simulink model "Non Augmented plant Nor Reference Non-constrained Input"  (R2013a)
settings: Solver=ode45  StartTime=0.0  StopTime=10.0  RelTol=1e-3
settings Model: Creator=G.force  LastModifiedBy=G.force

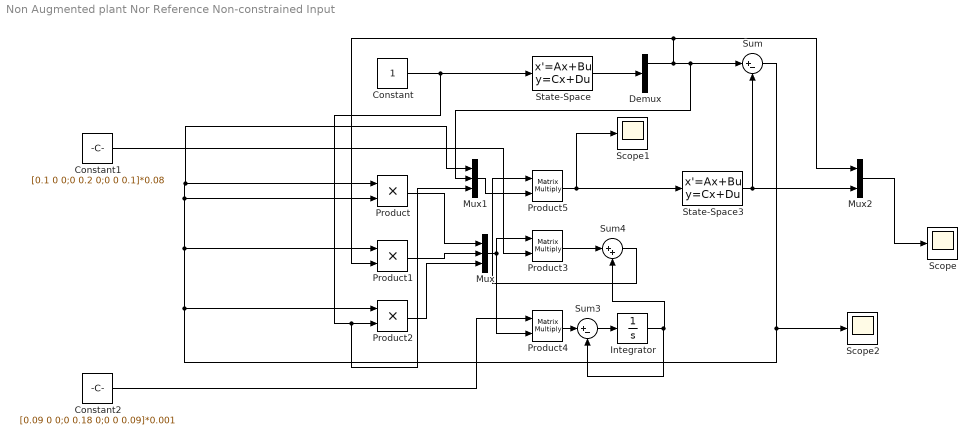
== system Non Augmented plant Nor Reference Non-constrained Input ==
  Constant : Constant
  Constant1 : Constant  Value=[0.1 0 0;0 0.2 0;0 0 0.1]*0.08
  Constant2 : Constant  Value=[0.09 0 0;0 0.18 0;0 0 0.09]*0.001
  Demux : Demux  Outputs=2
  Integrator : Integrator  InitialCondition=[0.01 0.0208 1e-6]
  Mux : Mux  Inputs=3
  Mux1 : Mux  Inputs=3
  Mux2 : Mux  Inputs=2
  Product : Product
  Product1 : Product
  Product2 : Product
  Product3 : Product  Multiplication=Matrix(*)
  Product4 : Product  Multiplication=Matrix(*)
  Product5 : Product  Multiplication=Matrix(*)
  Scope : Scope
      settings: ShowLegends=on  TimeRange=4  YMin=-40  YMax=45  SaveName=sd  MaxDataPoints=100000
  Scope1 : Scope
      settings: TimeRange=10  YMin=-3e+12  YMax=3e+12  SaveName=Up
  Scope2 : Scope
      settings: ShowLegends=on  TimeRange=4  YMin=-40  YMax=45  SaveName=E  MaxDataPoints=50000
  State-Space : StateSpace  A=[-1 0;0 -1]  B=[1;1]  C=eye(2)  D=[0;0]  X0=[2 0]
  State-Space3 : StateSpace  A=[0 1;-2084.1 0]  B=[0;0.9999]*1e5  C=[1 0]  D=0
  Sum : Sum  Inputs=|+-
  Sum3 : Sum  Inputs=|+-
  Sum4 : Sum  Inputs=|++
  wires:
  Constant/1 -> Mux1/3, Product2/2, State-Space/1
  Sum/1 -> Scope2/1, Product2/1, Product1/1, Product/2, Product/1, Mux1/1
  Product/1 -> Mux/1
  Product1/1 -> Mux/2
  Product2/1 -> Mux/3
  Mux/1 -> Product3/1, Product4/2
  Constant1/1 -> Product3/2
  Constant2/1 -> Product4/1
  Product4/1 -> Sum3/1
  Sum3/1 -> Integrator/1
  Product3/1 -> Sum4/1
  Sum4/1 -> Product5/1
  Mux1/1 -> Product5/2
  Mux2/1 -> Scope/1
  Integrator/1 -> Sum3/2, Sum4/2
  State-Space3/1 -> Mux2/2, Sum/2
  Product5/1 -> Scope1/1, State-Space3/1
  State-Space/1 -> Demux/1
  Demux/1 -> Product1/2, Mux2/1, Mux1/2, Sum/1
